simulink model "model_problem7"  (R2020a)
settings: Solver=VariableStepAuto  StartTime=0.0  StopTime=10.0  RelTol=1e-3
settings Model: Creator=Prateek  LastModifiedBy=Prateek

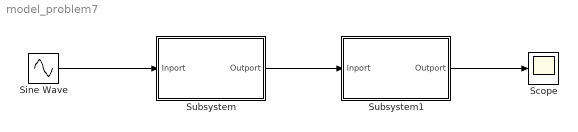
== system model_problem7 ==
  Scope : Scope
  Sine Wave : Sin  SampleTime=0
  Subsystem : Subsystem
  Subsystem1 : Subsystem
  wires:
  Sine Wave/1 -> Subsystem/1(Inport)
  Subsystem/1(Outport) -> Subsystem1/1(Inport)
  Subsystem1/1(Outport) -> Scope/1

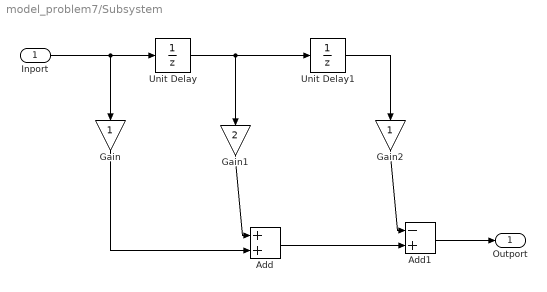
== system model_problem7/Subsystem ==
  Inport : Inport
  Add : Sum
  Add1 : Sum  Inputs=-+
  Gain : Gain
  Gain1 : Gain  Gain=2
  Gain2 : Gain
  Unit Delay : UnitDelay  SampleTime=-1  HasFrameUpgradeWarning=on
  Unit Delay1 : UnitDelay  SampleTime=-1  HasFrameUpgradeWarning=on
  Outport : Outport
  wires:
  Add1/1 -> Outport/1
  Unit Delay/1 -> Unit Delay1/1, Gain1/1
  Inport/1 -> Gain/1, Unit Delay/1
  Gain2/1 -> Add1/1
  Unit Delay1/1 -> Gain2/1
  Gain/1 -> Add/2
  Add/1 -> Add1/2
  Gain1/1 -> Add/1

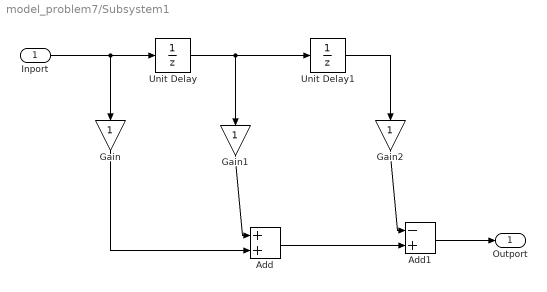
== system model_problem7/Subsystem1 ==
  Inport : Inport
  Add : Sum
  Add1 : Sum  Inputs=-+
  Gain : Gain
  Gain1 : Gain
  Gain2 : Gain
  Unit Delay : UnitDelay  SampleTime=-1  HasFrameUpgradeWarning=on
  Unit Delay1 : UnitDelay  SampleTime=-1  HasFrameUpgradeWarning=on
  Outport : Outport
  wires:
  Add1/1 -> Outport/1
  Unit Delay/1 -> Unit Delay1/1, Gain1/1
  Inport/1 -> Gain/1, Unit Delay/1
  Gain2/1 -> Add1/1
  Unit Delay1/1 -> Gain2/1
  Gain/1 -> Add/2
  Add/1 -> Add1/2
  Gain1/1 -> Add/1
